simulink model "q_qube2_oboe_sin2"  (R2020b)
settings: Solver=ode1  StartTime=0.0  StopTime=10  FixedStep=0.002  RelTol=1e-3  AbsTol=1e-6  EnableMultiTasking=on
values from neighbouring files (symbols this model uses):
  Festar1 = F1-L1*[1 0 0]    [TestDIST_EFFECT_DCmotor_zp(1).m]    (also in TestDIST_EFFECT_DCmotor_zp.m; lqr_DOB_2_5.mat = [-0.5  0.002  -0.000478501868071; -343.75  1  -0.47850186807; lqr_DOB_5.mat = [-0.5  0.002  -0.000478501868071; -343.75  1  -0.47850186807; lqr_DOB_8.mat = [-0.5  0.002  -0.000478501868071; -343.75  1  -0.47850186807)
  Gestar1 = [G1 L1]    [TestDIST_EFFECT_DCmotor_zp(1).m]    (also in TestDIST_EFFECT_DCmotor_zp.m; lqr_DOB_2_5.mat = [0.000478501868071  1.5; 0.478501868071  343.75; 0  -130.616; lqr_DOB_5.mat = [0.000478501868071  1.5; 0.478501868071  343.75; 0  -130.616; lqr_DOB_8.mat = [0.000478501868071  1.5; 0.478501868071  343.75; 0  -130.616)
  KK = dlqr(Fs,Gs,Q,R)    [TestDIST_EFFECT_DCmotor_zp(1).m]    (also in TestDIST_EFFECT_DCmotor_zp.m; lqr_DOB_2_5.mat = [27.9647466006 0.483496818901]; lqr_DOB_5.mat = [27.9647466006 0.483496818901]; lqr_DOB_8.mat = [27.9647466006 0.483496818901])
  Ts = 0.002    [TestDIST_EFFECT_DCmotor_zp(1).m]    (also in TestDIST_EFFECT_DCmotor_zp.m; lqr_DOB_2_5.mat; lqr_DOB_5.mat; lqr_DOB_8.mat)
undefined symbols (not defined in the file or in its folder): HIL, qc_get_step_size
libraries: quarc_library x4
settings Model: SimulationMode=external  ExtModeTrigDuration=5000000  Creator=MLevis  LastModifiedBy=marco
settings SolverCC: AutoScaleAbsTol=off  PositivePriorityOrder=on
settings DataIOCC: SaveFormat=Array  SignalLoggingSaveFormat=ModelDataLogs  ReturnWorkspaceOutputs=off
settings OptimizationCC: BlockReduction=off  BooleanDataType=off  OptimizeBlockIOStorage=off  BufferReuse=off  GlobalBufferReuse=off  ExpressionFolding=off  ExpressionDepthLimit=2147483647  LocalBlockOutputs=off  InitFltsAndDblsToZero=on  LifeSpan=inf  OptimizeDataStoreBuffers=off  BusAssignmentInplaceUpdate=off
settings DebuggingCC: SaveWithParameterizedLinksMsg=none  UnderspecifiedInitializationDetection=Classic  MergeDetectMultiDrivingBlocksExec=none  SignalResolutionControl=TryResolveAllWithWarning  MultiTaskDSMMsg=warning  MultiTaskCondExecSysMsg=none  FcnCallInpInsideContextMsg=warning  StateNameClashWarn=warning  SFUnexpectedBacktrackingDiag=warning  SFNoUnconditionalDefaultTransitionDiag=warning  SFExecutionAtInitializationDiag=none  ArithmeticOperatorsInVariantConditions=warning
settings HardwareCC: ProdBitPerPointer=32  ProdBitPerSizeT=32  ProdBitPerPtrDiffT=32  ProdLargestAtomicFloat=None  ProdIntDivRoundTo=Undefined  ProdEndianess=Unspecified  ProdWordSize=32  ProdHWDeviceType=32-bit Generic  TargetHWDeviceType=32-bit Generic
settings ModelReferenceCC: PropagateSignalLabelsOutOfModel=off
settings SFSimCC: SimUseLocalCustomCode=off  CustomCodeUndefinedFunction=UseInterfaceOnly
settings RTWCC: Description=QUARC Win64 Target  SystemTargetFile=quarc_win64.tlc  TemplateMakefile=quarc_default_tmf  RTWUseLocalCustomCode=off
settings CodeAppCC: StateflowObjectComments=on
settings STFCustomTargetCC: CPPClassGenCompliant=off
settings GRTTargetCC: TargetLangStandard=C89/C90 (ANSI)  ParMdlRefBuildCompliant=off  CompOptLevelCompliant=off  CombineOutputUpdateFcns=off  MatFileLogging=off  CPPClassGenCompliant=off  GRTInterface=on  UseToolchainInfoCompliant=off  ExtMode=on  ExtModeMexFile=quarc_comm
settings ConfigComp: CovMetricSettings=dw  CovSaveCumulativeToWorkspaceVar=on  CovSaveSingleToWorkspaceVar=on  CovExternalEMLEnable=off  CovSFcnEnable=off

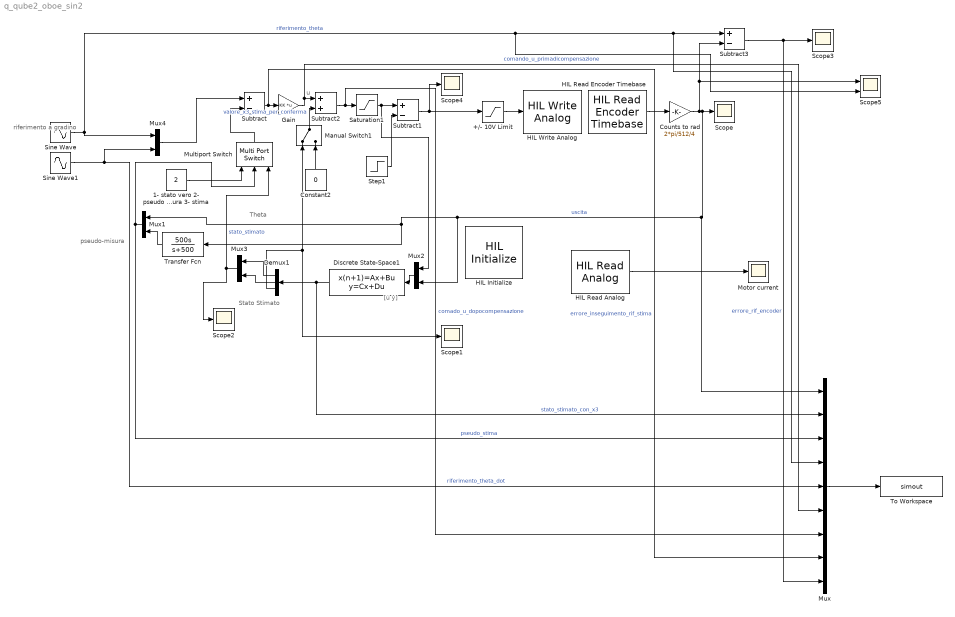
== system q_qube2_oboe_sin2 ==
  note: [u
      | y]
  note: Theta
  note: u
  note: Stato
      | Stimato
  note: pseudo-misura
  note: riferimento
      | a gradino
  +/- 10V Limit : Saturate  UpperLimit=20  LowerLimit=-20
  1- stato vero 2- pseudo misura 3- stima : Constant  Value=2
  Constant2 : Constant  Value=0
  Counts to rad : Gain  Gain=2*pi/512/4
  Demux1 : Demux  Outputs=3
  Discrete State-Space1 : DiscreteStateSpace  A=Festar1  B=Gestar1  C=eye(3)  D=[0 0; 0 0 ; 0 0]  InitialCondition=[0 0 0]'  SampleTime=Ts
  Gain : Gain  Gain=KK  Multiplication=Matrix(K*u)
  HIL Initialize : quarc_library/Data Acquisition/Generic/Configuration/HIL Initialize  Priority=-99  object_name=HIL-1  board_type=qube_servo2_usb  board_number=0  board_options=""  exclusive=off  active=off  hardware_clocks=[0]  clock_modes=[]  initial_clock_frequencies=[]  set_clock_params_at_start=off  set_clock_params_at_switch_in=off  set_clock_frequencies_at_start=off  set_clock_frequencies_at_switch_in=off  analog_input_channels=[0]  analog_input_configurations=[]  analog_input_maximums=3  analog_input_minimums=-3  set_analog_input_params_at_start=off  set_analog_input_params_at_switch_in=off  analog_output_channels=[0]  analog_output_maximums=15  analog_output_minimums=-15  initial_analog_outputs=[0]  final_analog_outputs=[0]  watchdog_analog_outputs=0  set_analog_output_params_at_start=off  set_analog_output_params_at_switch_in=off  set_analog_outputs_at_start=on  set_analog_outputs_at_switch_in=off  set_analog_outputs_at_terminate=on  set_analog_outputs_at_switch_out=off  set_analog_outputs_on_watchdog=on  digital_input_channels=[]  digital_output_channels=[0]  digital_output_configuration=[]  initial_digital_outputs=[1]  final_digital_outputs=[0]  watchdog_digital_outputs=[0]  set_digital_output_params_at_start=off  set_digital_output_params_at_switch_in=off  set_digital_outputs_at_start=on  set_digital_outputs_at_switch_in=off  set_digital_outputs_at_terminate=on  set_digital_outputs_at_switch_out=off  set_digital_outputs_on_watchdog=on  encoder_channels=[0:1]  quadrature=[4]  encoder_filter_frequency=[]  initial_encoder_counts=[0]  set_encoder_params_at_start=off  set_encoder_params_at_switch_in=off  set_encoder_counts_at_start=on  set_encoder_counts_at_switch_in=off  pwm_channels=[]  pwm_modes=[]  pwm_frequency=[]  pwm_configuration=[]  pwm_alignment=[]  pwm_polarity=[]  pwm_leading_deadband=[]  pwm_trailing_deadband=[]  initial_pwm_outputs=[]  final_pwm_outputs=[]  watchdog_pwm_outputs=[]  set_pwm_params_at_start=off  set_pwm_params_at_switch_in=off  set_pwm_outputs_at_start=off  set_pwm_outputs_at_switch_in=off  set_pwm_outputs_at_terminate=off  set_pwm_outputs_at_switch_out=off  set_pwm_outputs_on_watchdog=off  other_output_channels=[11000:11002]  initial_other_outputs=[0 1 0]  final_other_outputs=[1 0 0]  watchdog_other_outputs=[0 0 1]  set_other_outputs_at_start=on  set_other_outputs_at_switch_in=off  set_other_outputs_at_terminate=on  set_other_outputs_at_switch_out=off  set_other_outputs_on_watchdog=on
  HIL Read Analog : quarc_library/Data Acquisition/Generic/Immediate I//O/HIL Read Analog  object_name=HIL-1  channels=0  sample_time=qc_get_step_size  active=on  vector_output=off
  HIL Read Encoder Timebase : quarc_library/Data Acquisition/Generic/Timebases/HIL Read Encoder Timebase  object_name=HIL-1  clock=0  channels=0  active=on  vector_output=off  data_type_mode=Inherit via back propagation  data_type=double  overflow_mode=Error on overflow  samples_in_buffer=max(ceil(1/qc_get_step_size), 1)
  HIL Write Analog : quarc_library/Data Acquisition/Generic/Immediate I//O/HIL Write Analog  object_name=HIL-1  channels=0  sample_time=-1  active=off  vector_input=off
  Manual Switch1 : ManualSwitch
  Motor current : Scope
  Multiport Switch : MultiPortSwitch  Inputs=2
  Mux : Mux  Inputs=9
  Mux{1..4} (4 alike) : Mux  Inputs=2
  Saturation1 : Saturate  UpperLimit=20  LowerLimit=-20
  Scope{,1..4} (5 alike) : Scope
  Scope5 : Scope  NumInputPorts=2
  Sine Wave : Sin  SineType=Sample based  Samples=200  SampleTime=.002
  Sine Wave1 : Sin  SineType=Sample based  Amplitude=1*2*pi*2.5  Samples=200  SampleTime=.002  Offset=50
  Step1 : Step  Time=3  After=0  SampleTime=0
  Subtract : Sum  Inputs=+-
  Subtract1 : Sum  Inputs=+-
  Subtract2 : Sum
  Subtract3 : Sum  Inputs=+-
  To Workspace : ToWorkspace  VariableName=simout  SaveFormat=Structure With Time  SampleTime=-1
  Transfer Fcn : TransferFcn  Numerator=[500 0]  Denominator=[1 500]
  wires:
  HIL Read Encoder Timebase/1 -> Counts to rad/1
  Subtract1/1 -> +/- 10V Limit/1, Scope4/1
  +/- 10V Limit/1 -> HIL Write Analog/1
  HIL Read Analog/1 -> Motor current/1
  Constant2/1 -> Manual Switch1/2
  Demux1/1 -> Mux3/1
  Demux1/3 -> Scope1/1, Manual Switch1/1
  Demux1/2 -> Mux3/2
  Discrete State-Space1/1 -> Mux/2, Demux1/1  "stato_stimato_con_x3"
  1- stato vero 2- pseudo misura 3- stima/1 -> Multiport Switch/1
  Manual Switch1/1 -> Subtract2/2  "valore_x3_stima_per_conferma"
  Saturation1/1 -> Subtract1/1, Mux2/1
  Mux4/1 -> Subtract/1
  Multiport Switch/1 -> Subtract/2
  Mux2/1 -> Discrete State-Space1/1
  Transfer Fcn/1 -> Mux1/2
  Step1/1 -> Subtract1/2
  Subtract2/1 -> Mux/7, Saturation1/1  "comado_u_dopocompensazione"
  Subtract3/1 -> Mux/9, Scope3/1  "errore_rif_encoder"
  Mux/1 -> To Workspace/1
  Counts to rad/1 -> Scope5/1, Subtract3/2, Scope/1, Mux/1, Mux2/2, Transfer Fcn/1, Mux1/1  "uscita"
  Subtract/1 -> Mux/8, Gain/1  "errore_inseguimento_rif_stima"
  Mux3/1 -> Scope2/1, Multiport Switch/3  "stato_stimato"
  Gain/1 -> Mux/6, Subtract2/1  "comando_u_primadicompensazione"
  Mux1/1 -> Mux/3, Multiport Switch/2  "pseudo_stima"
  Sine Wave/1 -> Mux4/1, Scope5/2, Mux/4, Subtract3/1  "riferimento_theta"
  Sine Wave1/1 -> Mux/5, Mux4/2  "riferimento_theta_dot"
